simulink model "vrservo_simulink3d"  (R2020a)
settings: Solver=VariableStepAuto  StartTime=0.0  StopTime=100000  RelTol=1e-3
model workspace (MAT data in the model file):
  stepval = 1
undefined symbols (not defined in the file or in its folder): SetPointArea_Text
libraries: simulink x2, vrlib x2
settings Model: OrderedModelArguments=off  Creator=issa safar  LastModifiedBy=issa safar

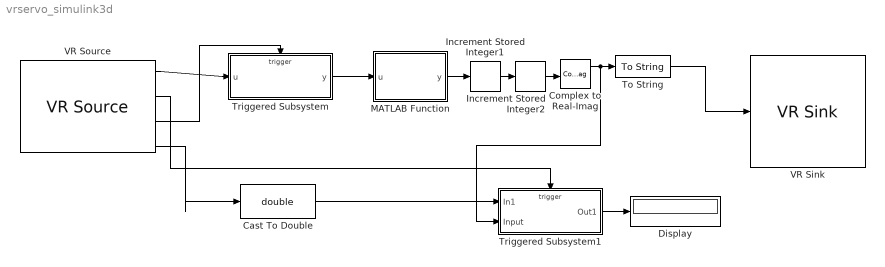
== system vrservo_simulink3d ==
  Cast To Double : DataTypeConversion  OutDataTypeStr=double
  Complex to Real-Imag : ComplexToRealImag
  Display : Display
  Increment Stored Integer1 : simulink/Additional Math & Discrete/Additional Math: Increment - Decrement/Increment Stored Integer
  Increment Stored Integer2 : simulink/Additional Math & Discrete/Additional Math: Increment - Decrement/Increment Stored Integer
  MATLAB Function : MATLAB Function  TreatAsAtomicUnit=on
  To String : ToString
  Triggered Subsystem : Subsystem  TreatAsAtomicUnit=on
  Triggered Subsystem1 : Subsystem  TreatAsAtomicUnit=on
  VR Sink : vrlib/VR Sink  InstantiateOnLoad=on  SampleTime=0.1  ViewEnable=on  RemoteChange=off  RemoteView=on  FieldsWritten=SetPointArea_Text.string.1.-1.1.char  WorldFileName=vrservo.x3d  WorldDescription=Virtual Control Panel  AutoView=on  VideoDimensions=[]  AllowVariableSize=off
  VR Source : vrlib/VR Source  InstantiateOnLoad=on  SampleTime=0.1  ViewEnable=on  RemoteChange=off  RemoteView=on  FieldsRead=SetPointArea_Text.string.1.1.1.char#Switch_1.Switch_State.1.1.1.logical#PushButton_1.Button_State.1.1.1.logical#Toggle_1.Toggle_State.1.1.1.logical  WorldFileName=vrservo.x3d  WorldDescription=Virtual Control Panel  AutoView=on  VideoDimensions=[]  AllowVariableSize=off
      settings: SourceProductBaseCode=SL
  wires:
  Complex to Real-Imag/1 -> Triggered Subsystem1/2(Input), To String/1
  Triggered Subsystem/1(y) -> MATLAB Function/1(u)
  MATLAB Function/1(y) -> Increment Stored Integer1/1
  Increment Stored Integer1/1 -> Increment Stored Integer2/1
  Increment Stored Integer2/1 -> Complex to Real-Imag/1
  VR Source/1 -> Triggered Subsystem/1(u)
  VR Source/3 -> Triggered Subsystem/Trigger
  To String/1 -> VR Sink/1
  VR Source/4 -> Cast To Double/1
  VR Source/2 -> Triggered Subsystem1/Trigger
  Cast To Double/1 -> Triggered Subsystem1/1(In1)
  Triggered Subsystem1/1(Out1) -> Display/1

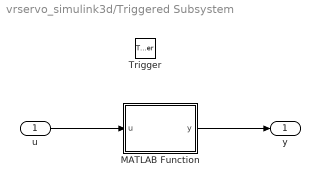
== system vrservo_simulink3d/Triggered Subsystem ==
  u : Inport
  Trigger : TriggerPort  VariantControl=Variant
  MATLAB Function : MATLAB Function  TreatAsAtomicUnit=on
  y : Outport
  wires:
  MATLAB Function/1(y) -> y/1
  u/1 -> MATLAB Function/1(u)

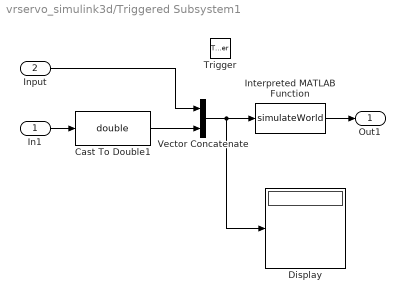
== system vrservo_simulink3d/Triggered Subsystem1 ==
  In1 : Inport
  Input : Inport  Port=2
  Trigger : TriggerPort  VariantControl=Variant
  Cast To Double1 : DataTypeConversion  OutDataTypeStr=double
  Display : Display
  Interpreted MATLAB Function : MATLABFcn  MATLABFcn=simulateWorld
  Vector Concatenate : Concatenate
  Out1 : Outport
  wires:
  In1/1 -> Cast To Double1/1
  Interpreted MATLAB Function/1 -> Out1/1
  Vector Concatenate/1 -> Display/1, Interpreted MATLAB Function/1
  Cast To Double1/1 -> Vector Concatenate/2
  Input/1 -> Vector Concatenate/1

== matlab function vrservo_simulink3d/Triggered Subsystem/MATLAB Function ==
  data: u input; y output
function y = fcn(u)

y = str2double(u);

== matlab function vrservo_simulink3d/MATLAB Function ==
  data: u input; y output
function y = fcn(u)
if(u==5||u==0)
    u=-1;
end
y = u;
